simulink model "hw7_sims"  (R2020b)
settings: Solver=VariableStepAuto  StartTime=0.0  StopTime=70  RelTol=1e-3
settings Model: Creator=abdullah  LastModifiedBy=abdullah

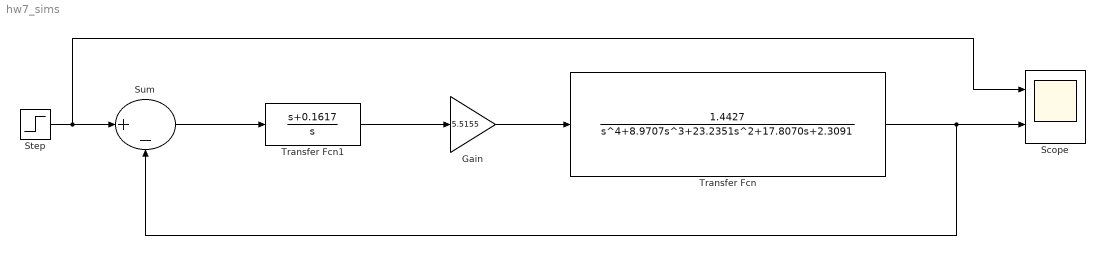
== system hw7_sims ==
  Gain : Gain  Gain=5.5155
  Scope : Scope  NumInputPorts=2
  Step : Step  SampleTime=0
  Sum : Sum  Inputs=|+-
  Transfer Fcn : TransferFcn  Numerator=[1.4427]  Denominator=[1 8.9707 23.2351 17.8070 2.3091]
  Transfer Fcn1 : TransferFcn  Numerator=[1 0.1617]  Denominator=[1 0]
  wires:
  Sum/1 -> Transfer Fcn1/1
  Transfer Fcn/1 -> Sum/2, Scope/2
  Step/1 -> Scope/1, Sum/1
  Gain/1 -> Transfer Fcn/1
  Transfer Fcn1/1 -> Gain/1
